simulink model "Supported_and_unsupported_combinations"  (Simulink 7.8)
settings: Solver=ode15s  StartTime=0.0  StopTime=inf  MaxStep=0.2  RelTol=1e-3
undefined symbols (not defined in the file): Engine, Engine1, Engine2, Engine3, Engine4, Engine5, Engine6, Engine7, Engine8, Engine9
libraries: sFunctionBlocks x32
(part 3 of 4)

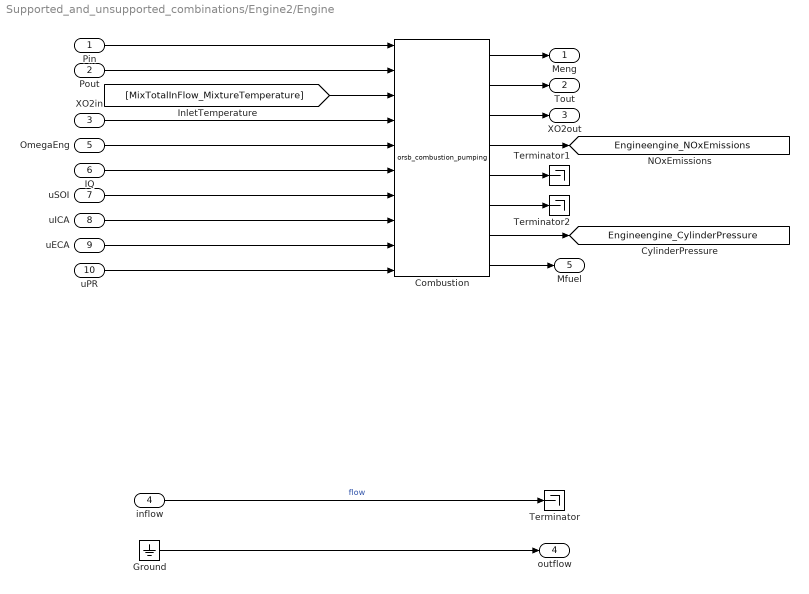
== system Supported_and_unsupported_combinations/Engine2/Engine ==
  Pin : Inport
  Pout : Inport  Port=2
  XO2in : Inport  Port=3
  inflow : Inport  Port=4
  OmegaEng : Inport  Port=5
  IQ : Inport  Port=6
  uSOI : Inport  Port=7
  uICA : Inport  Port=8
  uECA : Inport  Port=9
  uPR : Inport  Port=10
  Combustion : S-Function  FunctionName=orsb_combustion_pumping  Parameters=Displ, CompRatio, Ncyl, ValveMdl, TmpMdl, IgnitMdl, PressMdl, Cp, Cv, port_num_NOx, NOxMdl,  EnableBusSupport=off  mask(combustion_pumping){Displ=12.9, CompRatio=18, Ncyl=6, ValveMdl=[0.00961171539106083 -0.172384589641163], TmpMdl=[-0.025503095647334 0.175522235872159 0.0255043476751577 0.0373865335774022 0], IgnitMdl=[0.484351292851209 0.143524113288744 -0.055676015193126 -0.0109937044135945 -0.025686692856836], PressMdl=[5.48733176777509 -0.092135251339445 -0.0332005633970498 0.773921335537747], Cp=1500, Cv=1200, port_num_NOx=4, NOxMdl=[-0.0710772115732251 13.258266248882 2.53650929146028 -4.98871540780321 18.9690745540948 3.51983329140351 7.35640722696346 -29.5494146545499 -12.7663876549855 -0.0214097840965915 0.143608010417368 -1.21453634962735 0.541720620436424 -0.0774873942784366 -0.515304310267613]}
      mask prompts: Displ "displacement"; CompRatio "compression ratio"; Ncyl "number of cylinders"; ValveMdl "valve model"; TmpMdl "temperature model"; IgnitMdl "ignition model"; PressMdl "pressure model"; port_num_NOx "Model NOx output port number"; NOxMdl "NOx parameters"
      mask help: Combustion development
      mask TabNameString: geometry,geometry,geometry,thermodynamics,thermodynamics,thermodynamics,thermodynamics,thermodynamics,thermodynamics,NOx,NOx
      mask Display:
      | port_label('input', 1, 'Pi');
      | port_label('input', 2, 'Pe');
      | port_label('input', 3, 'Ti');
      | port_label('input', 4, 'O2i');
      | port_label('input', 5, 'Ne');
      | port_label('input', 6, 'iq');
      | port_label('input', 7, 'soi');
      | port_label('input', 8, 'ica');
      | port_label('input', 9, 'eca');
      | port_label('input', 10, 'Prail');
      | port_label('output', 1, 'M');
      | port_label('output', 2, 'Te');
      | port_label('output', 3, 'XO2e');
      | port_label('output', 4, 'NOx');
      | port_label('output', 5, 'lambda');
      | port_label('output', 6, 'phi_ign');
      | port_label('output', 7, 'Pcyl');
      | port_label('output', 8, 'Mf');
  Ground : Ground
  Terminator : Terminator
  Terminator1 : Terminator
  Terminator2 : Terminator
  Meng : Outport
  Tout : Outport  Port=2
  XO2out : Outport  Port=3
  outflow : Outport  Port=4
  Mfuel : Outport  Port=5
  tag scope: Engineengine_CylinderPressure=global, Engineengine_NOxEmissions=global
  wires:
  uSOI/1 -> Combustion/7
  [MixTotalInFlow_MixtureTemperature] -> Combustion/3
  Combustion/4 -> [Engineengine_NOxEmissions]
  XO2in/1 -> Combustion/4
  Combustion/3 -> XO2out/1
  Combustion/2 -> Tout/1
  Pout/1 -> Combustion/2
  Pin/1 -> Combustion/1
  OmegaEng/1 -> Combustion/5
  Ground/1 -> outflow/1
  inflow/1 -> Terminator/1  "flow"
  Combustion/1 -> Meng/1
  Combustion/5 -> Terminator1/1
  Combustion/6 -> Terminator2/1
  Combustion/7 -> [Engineengine_CylinderPressure]
  Combustion/8 -> Mfuel/1
  IQ/1 -> Combustion/6
  uICA/1 -> Combustion/8
  uECA/1 -> Combustion/9
  uPR/1 -> Combustion/10

== system Supported_and_unsupported_combinations/Engine2/ExhaustManifold ==
  Meng : Inport
  Tin : Inport  Port=2
  XO2in : Inport  Port=3
  inflow : Inport  Port=4
  Mfuel : Inport  Port=5
  Add4 : Sum
  AdiabaticManifoldXO2 : S-Function  FunctionName=orsb_reservoir_adiabatic_XO2  Parameters=V , R , Cp , pinit , Tinit , XO2init ,  EnableBusSupport=off  mask(reservoir adiabatic XO2 ){V=50, R=288.4, Cp=1135, pinit=247140, Tinit=720.22, XO2init=0.15}
      mask prompts: V "reservoir volume [l]"; R "gas constant [J/K/kg]"; Cp "fixed pressure spec heat [J/kg/K]"; pinit "initial pressure [Pa]"; Tinit "initial temperature [K]"; XO2init "initial oxygen mass fraction [-]"
      mask help: Adiabatic reservoir model with pressure, temperature, and oxygen mass fraction as internal states.
      mask TabNameString: General ,General ,General ,Initialization ,Initialization ,Initialization
      mask Display:
      | port_label('input', 1, 'min ');
      | port_label('input', 2, 'mout ');
      | port_label('input', 3, 'Tin ');
      | port_label('input', 4, 'O2min ');
      | port_label('output', 1, 'pout ');
      | port_label('output', 2, 'Tout ');
      | port_label('output', 3, 'XO2out ');
  Conversion_XO2_lambda : Fcn  Expr=u(1) / 0.231362 * (1 + 14.59) / (14.59 * (1 - u(1) / 0.231362))+1
  Product2 : Product  RndMeth=Zero
  Saturation : Saturate  UpperLimit=0.2313  LowerLimit=0
  Pout : Outport
  outflow : Outport  Port=2
  tag scope: EngineExhaustManifold_OutletLambda=global, EngineExhaustManifold_OutletOxygenFraction=global, EngineExhaustManifold_OutletPressure=global, EngineExhaustManifold_OutletTemperature=global
  wires:
  Conversion_XO2_lambda/1 -> [EngineExhaustManifold_OutletLambda]
  [FlowSplitterTotalOutFlow_Massflow] -> AdiabaticManifoldXO2/2
  Mfuel/1 -> Add4/1
  inflow/1 -> outflow/1  "flow"
  XO2in/1 -> Product2/2
  AdiabaticManifoldXO2/3 -> [EngineExhaustManifold_OutletOxygenFraction], Saturation/1
  Tin/1 -> AdiabaticManifoldXO2/3
  AdiabaticManifoldXO2/2 -> [EngineExhaustManifold_OutletTemperature]
  AdiabaticManifoldXO2/1 -> [EngineExhaustManifold_OutletPressure], Pout/1
  Meng/1 -> Add4/2
  Product2/1 -> AdiabaticManifoldXO2/4
  Add4/1 -> Product2/1, AdiabaticManifoldXO2/1
  Saturation/1 -> Conversion_XO2_lambda/1

== system Supported_and_unsupported_combinations/Engine2/IntakeManifold ==
  Mout : Inport
  inflow : Inport  Port=2
  IsothermalManifoldXO2 : S-Function  FunctionName=orsb_reservoir_isothermal_XO2  Parameters=V , R , Cp , pinit , XO2init ,  EnableBusSupport=off  mask(reservoir isothermal XO2 ){V=41.2801, R=288.4, Cp=1020, pinit=205590, XO2init=0.22}
      mask prompts: V "reservoir volume [l]"; R "gas constant [J/K/kg]"; Cp "fixed pressure spec heat [J/kg/K]"; pinit "initial pressure [Pa]"; XO2init "initial oxygen mass fraction [-]"
      mask help: Isothermal reservoir model with pressure and oxygen mass fraction as internal states.
      mask TabNameString: General ,General ,General ,Initialization ,Initialization
      mask Display:
      | port_label('input', 1, 'min ');
      | port_label('input', 2, 'mout ');
      | port_label('input', 3, 'Tin ');
      | port_label('input', 4, 'O2min ');
      | port_label('output', 1, 'pout ');
      | port_label('output', 2, 'XO2out ');
  Pim : Outport
  XO2out : Outport  Port=2
  outflow : Outport  Port=3
  tag scope: EngineIntakeManifold_OutletPressure=global
  wires:
  [MixTotalInFlow_MixtureTemperature] -> IsothermalManifoldXO2/3
  [MixTotalInFlow_OxygenFlow] -> IsothermalManifoldXO2/4
  [MixTotalInFlow_Massflow] -> IsothermalManifoldXO2/1
  inflow/1 -> outflow/1  "flow"
  IsothermalManifoldXO2/2 -> XO2out/1
  IsothermalManifoldXO2/1 -> [EngineIntakeManifold_OutletPressure], Pim/1
  Mout/1 -> IsothermalManifoldXO2/2

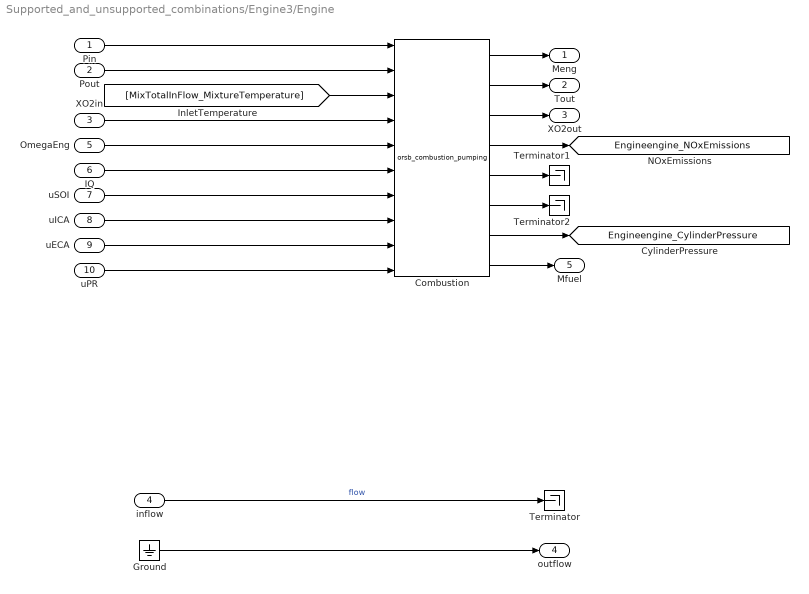
== system Supported_and_unsupported_combinations/Engine3/Engine ==
  Pin : Inport
  Pout : Inport  Port=2
  XO2in : Inport  Port=3
  inflow : Inport  Port=4
  OmegaEng : Inport  Port=5
  IQ : Inport  Port=6
  uSOI : Inport  Port=7
  uICA : Inport  Port=8
  uECA : Inport  Port=9
  uPR : Inport  Port=10
  Combustion : S-Function  FunctionName=orsb_combustion_pumping  Parameters=Displ, CompRatio, Ncyl, ValveMdl, TmpMdl, IgnitMdl, PressMdl, Cp, Cv, port_num_NOx, NOxMdl,  EnableBusSupport=off  mask(combustion_pumping){Displ=12.9, CompRatio=18, Ncyl=6, ValveMdl=[0.00961171539106083 -0.172384589641163], TmpMdl=[-0.025503095647334 0.175522235872159 0.0255043476751577 0.0373865335774022 0], IgnitMdl=[0.484351292851209 0.143524113288744 -0.055676015193126 -0.0109937044135945 -0.025686692856836], PressMdl=[5.48733176777509 -0.092135251339445 -0.0332005633970498 0.773921335537747], Cp=1500, Cv=1200, port_num_NOx=4, NOxMdl=[-0.0710772115732251 13.258266248882 2.53650929146028 -4.98871540780321 18.9690745540948 3.51983329140351 7.35640722696346 -29.5494146545499 -12.7663876549855 -0.0214097840965915 0.143608010417368 -1.21453634962735 0.541720620436424 -0.0774873942784366 -0.515304310267613]}
      mask prompts: Displ "displacement"; CompRatio "compression ratio"; Ncyl "number of cylinders"; ValveMdl "valve model"; TmpMdl "temperature model"; IgnitMdl "ignition model"; PressMdl "pressure model"; port_num_NOx "Model NOx output port number"; NOxMdl "NOx parameters"
      mask help: Combustion development
      mask TabNameString: geometry,geometry,geometry,thermodynamics,thermodynamics,thermodynamics,thermodynamics,thermodynamics,thermodynamics,NOx,NOx
      mask Display:
      | port_label('input', 1, 'Pi');
      | port_label('input', 2, 'Pe');
      | port_label('input', 3, 'Ti');
      | port_label('input', 4, 'O2i');
      | port_label('input', 5, 'Ne');
      | port_label('input', 6, 'iq');
      | port_label('input', 7, 'soi');
      | port_label('input', 8, 'ica');
      | port_label('input', 9, 'eca');
      | port_label('input', 10, 'Prail');
      | port_label('output', 1, 'M');
      | port_label('output', 2, 'Te');
      | port_label('output', 3, 'XO2e');
      | port_label('output', 4, 'NOx');
      | port_label('output', 5, 'lambda');
      | port_label('output', 6, 'phi_ign');
      | port_label('output', 7, 'Pcyl');
      | port_label('output', 8, 'Mf');
  Ground : Ground
  Terminator : Terminator
  Terminator1 : Terminator
  Terminator2 : Terminator
  Meng : Outport
  Tout : Outport  Port=2
  XO2out : Outport  Port=3
  outflow : Outport  Port=4
  Mfuel : Outport  Port=5
  tag scope: Engineengine_CylinderPressure=global, Engineengine_NOxEmissions=global
  wires:
  uPR/1 -> Combustion/10
  uECA/1 -> Combustion/9
  uICA/1 -> Combustion/8
  IQ/1 -> Combustion/6
  Combustion/8 -> Mfuel/1
  Combustion/7 -> [Engineengine_CylinderPressure]
  Combustion/6 -> Terminator2/1
  Combustion/5 -> Terminator1/1
  Combustion/1 -> Meng/1
  inflow/1 -> Terminator/1  "flow"
  Ground/1 -> outflow/1
  OmegaEng/1 -> Combustion/5
  Pin/1 -> Combustion/1
  Pout/1 -> Combustion/2
  Combustion/2 -> Tout/1
  Combustion/3 -> XO2out/1
  XO2in/1 -> Combustion/4
  Combustion/4 -> [Engineengine_NOxEmissions]
  [MixTotalInFlow_MixtureTemperature] -> Combustion/3
  uSOI/1 -> Combustion/7

== system Supported_and_unsupported_combinations/Engine3/ExhaustManifold ==
  Meng : Inport
  Tin : Inport  Port=2
  XO2in : Inport  Port=3
  inflow : Inport  Port=4
  Mfuel : Inport  Port=5
  Add4 : Sum
  AdiabaticManifoldXO2 : S-Function  FunctionName=orsb_reservoir_adiabatic_XO2  Parameters=V , R , Cp , pinit , Tinit , XO2init ,  EnableBusSupport=off  mask(reservoir adiabatic XO2 ){V=50, R=288.4, Cp=1135, pinit=247140, Tinit=720.22, XO2init=0.15}
      mask prompts: V "reservoir volume [l]"; R "gas constant [J/K/kg]"; Cp "fixed pressure spec heat [J/kg/K]"; pinit "initial pressure [Pa]"; Tinit "initial temperature [K]"; XO2init "initial oxygen mass fraction [-]"
      mask help: Adiabatic reservoir model with pressure, temperature, and oxygen mass fraction as internal states.
      mask TabNameString: General ,General ,General ,Initialization ,Initialization ,Initialization
      mask Display:
      | port_label('input', 1, 'min ');
      | port_label('input', 2, 'mout ');
      | port_label('input', 3, 'Tin ');
      | port_label('input', 4, 'O2min ');
      | port_label('output', 1, 'pout ');
      | port_label('output', 2, 'Tout ');
      | port_label('output', 3, 'XO2out ');
  Conversion_XO2_lambda : Fcn  Expr=u(1) / 0.231362 * (1 + 14.59) / (14.59 * (1 - u(1) / 0.231362))+1
  Product2 : Product  RndMeth=Zero
  Saturation : Saturate  UpperLimit=0.2313  LowerLimit=0
  Pout : Outport
  outflow : Outport  Port=2
  tag scope: EngineExhaustManifold_OutletLambda=global, EngineExhaustManifold_OutletOxygenFraction=global, EngineExhaustManifold_OutletPressure=global, EngineExhaustManifold_OutletTemperature=global
  wires:
  Saturation/1 -> Conversion_XO2_lambda/1
  Add4/1 -> AdiabaticManifoldXO2/1, Product2/1
  Product2/1 -> AdiabaticManifoldXO2/4
  Meng/1 -> Add4/2
  AdiabaticManifoldXO2/1 -> Pout/1, [EngineExhaustManifold_OutletPressure]
  AdiabaticManifoldXO2/2 -> [EngineExhaustManifold_OutletTemperature]
  Tin/1 -> AdiabaticManifoldXO2/3
  AdiabaticManifoldXO2/3 -> Saturation/1, [EngineExhaustManifold_OutletOxygenFraction]
  XO2in/1 -> Product2/2
  inflow/1 -> outflow/1  "flow"
  Mfuel/1 -> Add4/1
  [FlowSplitterTotalOutFlow_Massflow] -> AdiabaticManifoldXO2/2
  Conversion_XO2_lambda/1 -> [EngineExhaustManifold_OutletLambda]

== system Supported_and_unsupported_combinations/Engine3/IntakeManifold ==
  Mout : Inport
  inflow : Inport  Port=2
  IsothermalManifoldXO2 : S-Function  FunctionName=orsb_reservoir_isothermal_XO2  Parameters=V , R , Cp , pinit , XO2init ,  EnableBusSupport=off  mask(reservoir isothermal XO2 ){V=41.2801, R=288.4, Cp=1020, pinit=205590, XO2init=0.22}
      mask prompts: V "reservoir volume [l]"; R "gas constant [J/K/kg]"; Cp "fixed pressure spec heat [J/kg/K]"; pinit "initial pressure [Pa]"; XO2init "initial oxygen mass fraction [-]"
      mask help: Isothermal reservoir model with pressure and oxygen mass fraction as internal states.
      mask TabNameString: General ,General ,General ,Initialization ,Initialization
      mask Display:
      | port_label('input', 1, 'min ');
      | port_label('input', 2, 'mout ');
      | port_label('input', 3, 'Tin ');
      | port_label('input', 4, 'O2min ');
      | port_label('output', 1, 'pout ');
      | port_label('output', 2, 'XO2out ');
  Pim : Outport
  XO2out : Outport  Port=2
  outflow : Outport  Port=3
  tag scope: EngineIntakeManifold_OutletPressure=global
  wires:
  Mout/1 -> IsothermalManifoldXO2/2
  IsothermalManifoldXO2/1 -> Pim/1, [EngineIntakeManifold_OutletPressure]
  IsothermalManifoldXO2/2 -> XO2out/1
  inflow/1 -> outflow/1  "flow"
  [MixTotalInFlow_Massflow] -> IsothermalManifoldXO2/1
  [MixTotalInFlow_OxygenFlow] -> IsothermalManifoldXO2/4
  [MixTotalInFlow_MixtureTemperature] -> IsothermalManifoldXO2/3

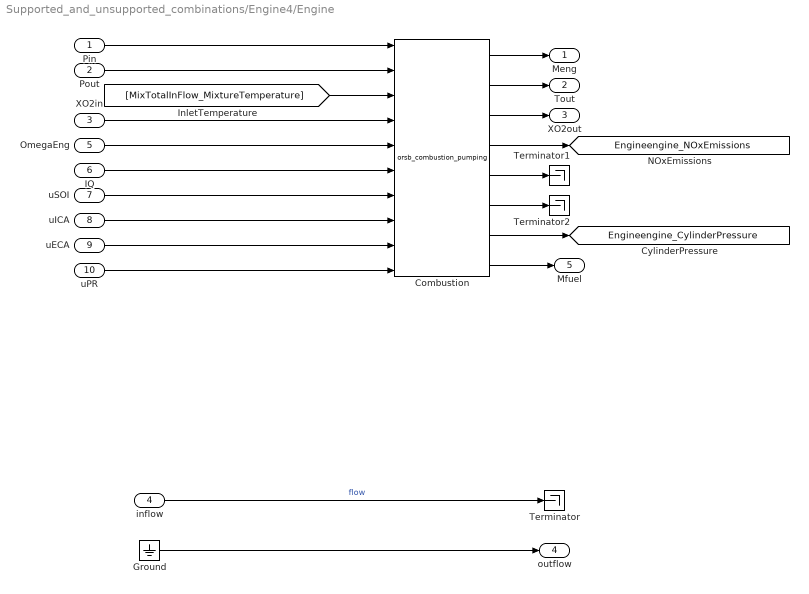
== system Supported_and_unsupported_combinations/Engine4/Engine ==
  Pin : Inport
  Pout : Inport  Port=2
  XO2in : Inport  Port=3
  inflow : Inport  Port=4
  OmegaEng : Inport  Port=5
  IQ : Inport  Port=6
  uSOI : Inport  Port=7
  uICA : Inport  Port=8
  uECA : Inport  Port=9
  uPR : Inport  Port=10
  Combustion : S-Function  FunctionName=orsb_combustion_pumping  Parameters=Displ, CompRatio, Ncyl, ValveMdl, TmpMdl, IgnitMdl, PressMdl, Cp, Cv, port_num_NOx, NOxMdl,  EnableBusSupport=off  mask(combustion_pumping){Displ=12.9, CompRatio=18, Ncyl=6, ValveMdl=[0.00961171539106083 -0.172384589641163], TmpMdl=[-0.025503095647334 0.175522235872159 0.0255043476751577 0.0373865335774022 0], IgnitMdl=[0.484351292851209 0.143524113288744 -0.055676015193126 -0.0109937044135945 -0.025686692856836], PressMdl=[5.48733176777509 -0.092135251339445 -0.0332005633970498 0.773921335537747], Cp=1500, Cv=1200, port_num_NOx=4, NOxMdl=[-0.0710772115732251 13.258266248882 2.53650929146028 -4.98871540780321 18.9690745540948 3.51983329140351 7.35640722696346 -29.5494146545499 -12.7663876549855 -0.0214097840965915 0.143608010417368 -1.21453634962735 0.541720620436424 -0.0774873942784366 -0.515304310267613]}
      mask prompts: Displ "displacement"; CompRatio "compression ratio"; Ncyl "number of cylinders"; ValveMdl "valve model"; TmpMdl "temperature model"; IgnitMdl "ignition model"; PressMdl "pressure model"; port_num_NOx "Model NOx output port number"; NOxMdl "NOx parameters"
      mask help: Combustion development
      mask TabNameString: geometry,geometry,geometry,thermodynamics,thermodynamics,thermodynamics,thermodynamics,thermodynamics,thermodynamics,NOx,NOx
      mask Display:
      | port_label('input', 1, 'Pi');
      | port_label('input', 2, 'Pe');
      | port_label('input', 3, 'Ti');
      | port_label('input', 4, 'O2i');
      | port_label('input', 5, 'Ne');
      | port_label('input', 6, 'iq');
      | port_label('input', 7, 'soi');
      | port_label('input', 8, 'ica');
      | port_label('input', 9, 'eca');
      | port_label('input', 10, 'Prail');
      | port_label('output', 1, 'M');
      | port_label('output', 2, 'Te');
      | port_label('output', 3, 'XO2e');
      | port_label('output', 4, 'NOx');
      | port_label('output', 5, 'lambda');
      | port_label('output', 6, 'phi_ign');
      | port_label('output', 7, 'Pcyl');
      | port_label('output', 8, 'Mf');
  Ground : Ground
  Terminator : Terminator
  Terminator1 : Terminator
  Terminator2 : Terminator
  Meng : Outport
  Tout : Outport  Port=2
  XO2out : Outport  Port=3
  outflow : Outport  Port=4
  Mfuel : Outport  Port=5
  tag scope: Engineengine_CylinderPressure=global, Engineengine_NOxEmissions=global
  wires:
  uSOI/1 -> Combustion/7
  [MixTotalInFlow_MixtureTemperature] -> Combustion/3
  Combustion/4 -> [Engineengine_NOxEmissions]
  XO2in/1 -> Combustion/4
  Combustion/3 -> XO2out/1
  Combustion/2 -> Tout/1
  Pout/1 -> Combustion/2
  Pin/1 -> Combustion/1
  OmegaEng/1 -> Combustion/5
  Ground/1 -> outflow/1
  inflow/1 -> Terminator/1  "flow"
  Combustion/1 -> Meng/1
  Combustion/5 -> Terminator1/1
  Combustion/6 -> Terminator2/1
  Combustion/7 -> [Engineengine_CylinderPressure]
  Combustion/8 -> Mfuel/1
  IQ/1 -> Combustion/6
  uICA/1 -> Combustion/8
  uECA/1 -> Combustion/9
  uPR/1 -> Combustion/10

== system Supported_and_unsupported_combinations/Engine4/ExhaustManifold ==
  Meng : Inport
  Tin : Inport  Port=2
  XO2in : Inport  Port=3
  inflow : Inport  Port=4
  Mfuel : Inport  Port=5
  Add4 : Sum
  AdiabaticManifoldXO2 : S-Function  FunctionName=orsb_reservoir_adiabatic_XO2  Parameters=V , R , Cp , pinit , Tinit , XO2init ,  EnableBusSupport=off  mask(reservoir adiabatic XO2 ){V=50, R=288.4, Cp=1135, pinit=247140, Tinit=720.22, XO2init=0.15}
      mask prompts: V "reservoir volume [l]"; R "gas constant [J/K/kg]"; Cp "fixed pressure spec heat [J/kg/K]"; pinit "initial pressure [Pa]"; Tinit "initial temperature [K]"; XO2init "initial oxygen mass fraction [-]"
      mask help: Adiabatic reservoir model with pressure, temperature, and oxygen mass fraction as internal states.
      mask TabNameString: General ,General ,General ,Initialization ,Initialization ,Initialization
      mask Display:
      | port_label('input', 1, 'min ');
      | port_label('input', 2, 'mout ');
      | port_label('input', 3, 'Tin ');
      | port_label('input', 4, 'O2min ');
      | port_label('output', 1, 'pout ');
      | port_label('output', 2, 'Tout ');
      | port_label('output', 3, 'XO2out ');
  Conversion_XO2_lambda : Fcn  Expr=u(1) / 0.231362 * (1 + 14.59) / (14.59 * (1 - u(1) / 0.231362))+1
  Product2 : Product  RndMeth=Zero
  Saturation : Saturate  UpperLimit=0.2313  LowerLimit=0
  Pout : Outport
  outflow : Outport  Port=2
  tag scope: EngineExhaustManifold_OutletLambda=global, EngineExhaustManifold_OutletOxygenFraction=global, EngineExhaustManifold_OutletPressure=global, EngineExhaustManifold_OutletTemperature=global
  wires:
  Conversion_XO2_lambda/1 -> [EngineExhaustManifold_OutletLambda]
  [FlowSplitterTotalOutFlow_Massflow] -> AdiabaticManifoldXO2/2
  Mfuel/1 -> Add4/1
  inflow/1 -> outflow/1  "flow"
  XO2in/1 -> Product2/2
  AdiabaticManifoldXO2/3 -> [EngineExhaustManifold_OutletOxygenFraction], Saturation/1
  Tin/1 -> AdiabaticManifoldXO2/3
  AdiabaticManifoldXO2/2 -> [EngineExhaustManifold_OutletTemperature]
  AdiabaticManifoldXO2/1 -> [EngineExhaustManifold_OutletPressure], Pout/1
  Meng/1 -> Add4/2
  Product2/1 -> AdiabaticManifoldXO2/4
  Add4/1 -> Product2/1, AdiabaticManifoldXO2/1
  Saturation/1 -> Conversion_XO2_lambda/1

== system Supported_and_unsupported_combinations/Engine4/IntakeManifold ==
  Mout : Inport
  inflow : Inport  Port=2
  IsothermalManifoldXO2 : S-Function  FunctionName=orsb_reservoir_isothermal_XO2  Parameters=V , R , Cp , pinit , XO2init ,  EnableBusSupport=off  mask(reservoir isothermal XO2 ){V=41.2801, R=288.4, Cp=1020, pinit=205590, XO2init=0.22}
      mask prompts: V "reservoir volume [l]"; R "gas constant [J/K/kg]"; Cp "fixed pressure spec heat [J/kg/K]"; pinit "initial pressure [Pa]"; XO2init "initial oxygen mass fraction [-]"
      mask help: Isothermal reservoir model with pressure and oxygen mass fraction as internal states.
      mask TabNameString: General ,General ,General ,Initialization ,Initialization
      mask Display:
      | port_label('input', 1, 'min ');
      | port_label('input', 2, 'mout ');
      | port_label('input', 3, 'Tin ');
      | port_label('input', 4, 'O2min ');
      | port_label('output', 1, 'pout ');
      | port_label('output', 2, 'XO2out ');
  Pim : Outport
  XO2out : Outport  Port=2
  outflow : Outport  Port=3
  tag scope: EngineIntakeManifold_OutletPressure=global
  wires:
  [MixTotalInFlow_MixtureTemperature] -> IsothermalManifoldXO2/3
  [MixTotalInFlow_OxygenFlow] -> IsothermalManifoldXO2/4
  [MixTotalInFlow_Massflow] -> IsothermalManifoldXO2/1
  inflow/1 -> outflow/1  "flow"
  IsothermalManifoldXO2/2 -> XO2out/1
  IsothermalManifoldXO2/1 -> [EngineIntakeManifold_OutletPressure], Pim/1
  Mout/1 -> IsothermalManifoldXO2/2

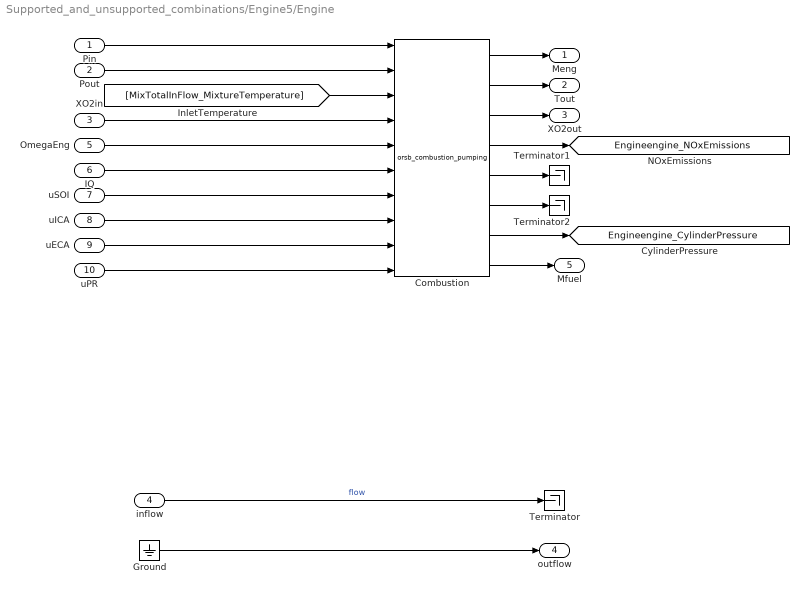
== system Supported_and_unsupported_combinations/Engine5/Engine ==
  Pin : Inport
  Pout : Inport  Port=2
  XO2in : Inport  Port=3
  inflow : Inport  Port=4
  OmegaEng : Inport  Port=5
  IQ : Inport  Port=6
  uSOI : Inport  Port=7
  uICA : Inport  Port=8
  uECA : Inport  Port=9
  uPR : Inport  Port=10
  Combustion : S-Function  FunctionName=orsb_combustion_pumping  Parameters=Displ, CompRatio, Ncyl, ValveMdl, TmpMdl, IgnitMdl, PressMdl, Cp, Cv, port_num_NOx, NOxMdl,  EnableBusSupport=off  mask(combustion_pumping){Displ=12.9, CompRatio=18, Ncyl=6, ValveMdl=[0.00961171539106083 -0.172384589641163], TmpMdl=[-0.025503095647334 0.175522235872159 0.0255043476751577 0.0373865335774022 0], IgnitMdl=[0.484351292851209 0.143524113288744 -0.055676015193126 -0.0109937044135945 -0.025686692856836], PressMdl=[5.48733176777509 -0.092135251339445 -0.0332005633970498 0.773921335537747], Cp=1500, Cv=1200, port_num_NOx=4, NOxMdl=[-0.0710772115732251 13.258266248882 2.53650929146028 -4.98871540780321 18.9690745540948 3.51983329140351 7.35640722696346 -29.5494146545499 -12.7663876549855 -0.0214097840965915 0.143608010417368 -1.21453634962735 0.541720620436424 -0.0774873942784366 -0.515304310267613]}
      mask prompts: Displ "displacement"; CompRatio "compression ratio"; Ncyl "number of cylinders"; ValveMdl "valve model"; TmpMdl "temperature model"; IgnitMdl "ignition model"; PressMdl "pressure model"; port_num_NOx "Model NOx output port number"; NOxMdl "NOx parameters"
      mask help: Combustion development
      mask TabNameString: geometry,geometry,geometry,thermodynamics,thermodynamics,thermodynamics,thermodynamics,thermodynamics,thermodynamics,NOx,NOx
      mask Display:
      | port_label('input', 1, 'Pi');
      | port_label('input', 2, 'Pe');
      | port_label('input', 3, 'Ti');
      | port_label('input', 4, 'O2i');
      | port_label('input', 5, 'Ne');
      | port_label('input', 6, 'iq');
      | port_label('input', 7, 'soi');
      | port_label('input', 8, 'ica');
      | port_label('input', 9, 'eca');
      | port_label('input', 10, 'Prail');
      | port_label('output', 1, 'M');
      | port_label('output', 2, 'Te');
      | port_label('output', 3, 'XO2e');
      | port_label('output', 4, 'NOx');
      | port_label('output', 5, 'lambda');
      | port_label('output', 6, 'phi_ign');
      | port_label('output', 7, 'Pcyl');
      | port_label('output', 8, 'Mf');
  Ground : Ground
  Terminator : Terminator
  Terminator1 : Terminator
  Terminator2 : Terminator
  Meng : Outport
  Tout : Outport  Port=2
  XO2out : Outport  Port=3
  outflow : Outport  Port=4
  Mfuel : Outport  Port=5
  tag scope: Engineengine_CylinderPressure=global, Engineengine_NOxEmissions=global
  wires:
  uPR/1 -> Combustion/10
  uECA/1 -> Combustion/9
  uICA/1 -> Combustion/8
  IQ/1 -> Combustion/6
  Combustion/8 -> Mfuel/1
  Combustion/7 -> [Engineengine_CylinderPressure]
  Combustion/6 -> Terminator2/1
  Combustion/5 -> Terminator1/1
  Combustion/1 -> Meng/1
  inflow/1 -> Terminator/1  "flow"
  Ground/1 -> outflow/1
  OmegaEng/1 -> Combustion/5
  Pin/1 -> Combustion/1
  Pout/1 -> Combustion/2
  Combustion/2 -> Tout/1
  Combustion/3 -> XO2out/1
  XO2in/1 -> Combustion/4
  Combustion/4 -> [Engineengine_NOxEmissions]
  [MixTotalInFlow_MixtureTemperature] -> Combustion/3
  uSOI/1 -> Combustion/7

== system Supported_and_unsupported_combinations/Engine5/ExhaustManifold ==
  Meng : Inport
  Tin : Inport  Port=2
  XO2in : Inport  Port=3
  inflow : Inport  Port=4
  Mfuel : Inport  Port=5
  Add4 : Sum
  AdiabaticManifoldXO2 : S-Function  FunctionName=orsb_reservoir_adiabatic_XO2  Parameters=V , R , Cp , pinit , Tinit , XO2init ,  EnableBusSupport=off  mask(reservoir adiabatic XO2 ){V=50, R=288.4, Cp=1135, pinit=247140, Tinit=720.22, XO2init=0.15}
      mask prompts: V "reservoir volume [l]"; R "gas constant [J/K/kg]"; Cp "fixed pressure spec heat [J/kg/K]"; pinit "initial pressure [Pa]"; Tinit "initial temperature [K]"; XO2init "initial oxygen mass fraction [-]"
      mask help: Adiabatic reservoir model with pressure, temperature, and oxygen mass fraction as internal states.
      mask TabNameString: General ,General ,General ,Initialization ,Initialization ,Initialization
      mask Display:
      | port_label('input', 1, 'min ');
      | port_label('input', 2, 'mout ');
      | port_label('input', 3, 'Tin ');
      | port_label('input', 4, 'O2min ');
      | port_label('output', 1, 'pout ');
      | port_label('output', 2, 'Tout ');
      | port_label('output', 3, 'XO2out ');
  Conversion_XO2_lambda : Fcn  Expr=u(1) / 0.231362 * (1 + 14.59) / (14.59 * (1 - u(1) / 0.231362))+1
  Product2 : Product  RndMeth=Zero
  Saturation : Saturate  UpperLimit=0.2313  LowerLimit=0
  Pout : Outport
  outflow : Outport  Port=2
  tag scope: EngineExhaustManifold_OutletLambda=global, EngineExhaustManifold_OutletOxygenFraction=global, EngineExhaustManifold_OutletPressure=global, EngineExhaustManifold_OutletTemperature=global
  wires:
  Saturation/1 -> Conversion_XO2_lambda/1
  Add4/1 -> AdiabaticManifoldXO2/1, Product2/1
  Product2/1 -> AdiabaticManifoldXO2/4
  Meng/1 -> Add4/2
  AdiabaticManifoldXO2/1 -> Pout/1, [EngineExhaustManifold_OutletPressure]
  AdiabaticManifoldXO2/2 -> [EngineExhaustManifold_OutletTemperature]
  Tin/1 -> AdiabaticManifoldXO2/3
  AdiabaticManifoldXO2/3 -> Saturation/1, [EngineExhaustManifold_OutletOxygenFraction]
  XO2in/1 -> Product2/2
  inflow/1 -> outflow/1  "flow"
  Mfuel/1 -> Add4/1
  [FlowSplitterTotalOutFlow_Massflow] -> AdiabaticManifoldXO2/2
  Conversion_XO2_lambda/1 -> [EngineExhaustManifold_OutletLambda]

== system Supported_and_unsupported_combinations/Engine5/IntakeManifold ==
  Mout : Inport
  inflow : Inport  Port=2
  IsothermalManifoldXO2 : S-Function  FunctionName=orsb_reservoir_isothermal_XO2  Parameters=V , R , Cp , pinit , XO2init ,  EnableBusSupport=off  mask(reservoir isothermal XO2 ){V=41.2801, R=288.4, Cp=1020, pinit=205590, XO2init=0.22}
      mask prompts: V "reservoir volume [l]"; R "gas constant [J/K/kg]"; Cp "fixed pressure spec heat [J/kg/K]"; pinit "initial pressure [Pa]"; XO2init "initial oxygen mass fraction [-]"
      mask help: Isothermal reservoir model with pressure and oxygen mass fraction as internal states.
      mask TabNameString: General ,General ,General ,Initialization ,Initialization
      mask Display:
      | port_label('input', 1, 'min ');
      | port_label('input', 2, 'mout ');
      | port_label('input', 3, 'Tin ');
      | port_label('input', 4, 'O2min ');
      | port_label('output', 1, 'pout ');
      | port_label('output', 2, 'XO2out ');
  Pim : Outport
  XO2out : Outport  Port=2
  outflow : Outport  Port=3
  tag scope: EngineIntakeManifold_OutletPressure=global
  wires:
  Mout/1 -> IsothermalManifoldXO2/2
  IsothermalManifoldXO2/1 -> Pim/1, [EngineIntakeManifold_OutletPressure]
  IsothermalManifoldXO2/2 -> XO2out/1
  inflow/1 -> outflow/1  "flow"
  [MixTotalInFlow_Massflow] -> IsothermalManifoldXO2/1
  [MixTotalInFlow_OxygenFlow] -> IsothermalManifoldXO2/4
  [MixTotalInFlow_MixtureTemperature] -> IsothermalManifoldXO2/3

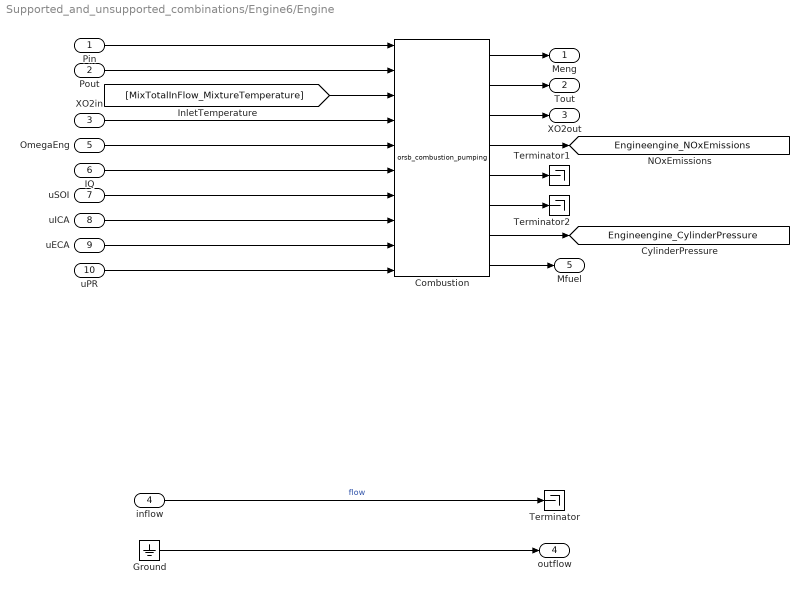
== system Supported_and_unsupported_combinations/Engine6/Engine ==
  Pin : Inport
  Pout : Inport  Port=2
  XO2in : Inport  Port=3
  inflow : Inport  Port=4
  OmegaEng : Inport  Port=5
  IQ : Inport  Port=6
  uSOI : Inport  Port=7
  uICA : Inport  Port=8
  uECA : Inport  Port=9
  uPR : Inport  Port=10
  Combustion : S-Function  FunctionName=orsb_combustion_pumping  Parameters=Displ, CompRatio, Ncyl, ValveMdl, TmpMdl, IgnitMdl, PressMdl, Cp, Cv, port_num_NOx, NOxMdl,  EnableBusSupport=off  mask(combustion_pumping){Displ=12.9, CompRatio=18, Ncyl=6, ValveMdl=[0.00961171539106083 -0.172384589641163], TmpMdl=[-0.025503095647334 0.175522235872159 0.0255043476751577 0.0373865335774022 0], IgnitMdl=[0.484351292851209 0.143524113288744 -0.055676015193126 -0.0109937044135945 -0.025686692856836], PressMdl=[5.48733176777509 -0.092135251339445 -0.0332005633970498 0.773921335537747], Cp=1500, Cv=1200, port_num_NOx=4, NOxMdl=[-0.0710772115732251 13.258266248882 2.53650929146028 -4.98871540780321 18.9690745540948 3.51983329140351 7.35640722696346 -29.5494146545499 -12.7663876549855 -0.0214097840965915 0.143608010417368 -1.21453634962735 0.541720620436424 -0.0774873942784366 -0.515304310267613]}
      mask prompts: Displ "displacement"; CompRatio "compression ratio"; Ncyl "number of cylinders"; ValveMdl "valve model"; TmpMdl "temperature model"; IgnitMdl "ignition model"; PressMdl "pressure model"; port_num_NOx "Model NOx output port number"; NOxMdl "NOx parameters"
      mask help: Combustion development
      mask TabNameString: geometry,geometry,geometry,thermodynamics,thermodynamics,thermodynamics,thermodynamics,thermodynamics,thermodynamics,NOx,NOx
      mask Display:
      | port_label('input', 1, 'Pi');
      | port_label('input', 2, 'Pe');
      | port_label('input', 3, 'Ti');
      | port_label('input', 4, 'O2i');
      | port_label('input', 5, 'Ne');
      | port_label('input', 6, 'iq');
      | port_label('input', 7, 'soi');
      | port_label('input', 8, 'ica');
      | port_label('input', 9, 'eca');
      | port_label('input', 10, 'Prail');
      | port_label('output', 1, 'M');
      | port_label('output', 2, 'Te');
      | port_label('output', 3, 'XO2e');
      | port_label('output', 4, 'NOx');
      | port_label('output', 5, 'lambda');
      | port_label('output', 6, 'phi_ign');
      | port_label('output', 7, 'Pcyl');
      | port_label('output', 8, 'Mf');
  Ground : Ground
  Terminator : Terminator
  Terminator1 : Terminator
  Terminator2 : Terminator
  Meng : Outport
  Tout : Outport  Port=2
  XO2out : Outport  Port=3
  outflow : Outport  Port=4
  Mfuel : Outport  Port=5
  tag scope: Engineengine_CylinderPressure=global, Engineengine_NOxEmissions=global
  wires:
  uPR/1 -> Combustion/10
  uECA/1 -> Combustion/9
  uICA/1 -> Combustion/8
  IQ/1 -> Combustion/6
  Combustion/8 -> Mfuel/1
  Combustion/7 -> [Engineengine_CylinderPressure]
  Combustion/6 -> Terminator2/1
  Combustion/5 -> Terminator1/1
  Combustion/1 -> Meng/1
  inflow/1 -> Terminator/1  "flow"
  Ground/1 -> outflow/1
  OmegaEng/1 -> Combustion/5
  Pin/1 -> Combustion/1
  Pout/1 -> Combustion/2
  Combustion/2 -> Tout/1
  Combustion/3 -> XO2out/1
  XO2in/1 -> Combustion/4
  Combustion/4 -> [Engineengine_NOxEmissions]
  [MixTotalInFlow_MixtureTemperature] -> Combustion/3
  uSOI/1 -> Combustion/7

== system Supported_and_unsupported_combinations/Engine6/ExhaustManifold ==
  Meng : Inport
  Tin : Inport  Port=2
  XO2in : Inport  Port=3
  inflow : Inport  Port=4
  Mfuel : Inport  Port=5
  Add4 : Sum
  AdiabaticManifoldXO2 : S-Function  FunctionName=orsb_reservoir_adiabatic_XO2  Parameters=V , R , Cp , pinit , Tinit , XO2init ,  EnableBusSupport=off  mask(reservoir adiabatic XO2 ){V=50, R=288.4, Cp=1135, pinit=247140, Tinit=720.22, XO2init=0.15}
      mask prompts: V "reservoir volume [l]"; R "gas constant [J/K/kg]"; Cp "fixed pressure spec heat [J/kg/K]"; pinit "initial pressure [Pa]"; Tinit "initial temperature [K]"; XO2init "initial oxygen mass fraction [-]"
      mask help: Adiabatic reservoir model with pressure, temperature, and oxygen mass fraction as internal states.
      mask TabNameString: General ,General ,General ,Initialization ,Initialization ,Initialization
      mask Display:
      | port_label('input', 1, 'min ');
      | port_label('input', 2, 'mout ');
      | port_label('input', 3, 'Tin ');
      | port_label('input', 4, 'O2min ');
      | port_label('output', 1, 'pout ');
      | port_label('output', 2, 'Tout ');
      | port_label('output', 3, 'XO2out ');
  Conversion_XO2_lambda : Fcn  Expr=u(1) / 0.231362 * (1 + 14.59) / (14.59 * (1 - u(1) / 0.231362))+1
  Product2 : Product  RndMeth=Zero
  Saturation : Saturate  UpperLimit=0.2313  LowerLimit=0
  Pout : Outport
  outflow : Outport  Port=2
  tag scope: EngineExhaustManifold_OutletLambda=global, EngineExhaustManifold_OutletOxygenFraction=global, EngineExhaustManifold_OutletPressure=global, EngineExhaustManifold_OutletTemperature=global
  wires:
  Saturation/1 -> Conversion_XO2_lambda/1
  Add4/1 -> AdiabaticManifoldXO2/1, Product2/1
  Product2/1 -> AdiabaticManifoldXO2/4
  Meng/1 -> Add4/2
  AdiabaticManifoldXO2/1 -> Pout/1, [EngineExhaustManifold_OutletPressure]
  AdiabaticManifoldXO2/2 -> [EngineExhaustManifold_OutletTemperature]
  Tin/1 -> AdiabaticManifoldXO2/3
  AdiabaticManifoldXO2/3 -> Saturation/1, [EngineExhaustManifold_OutletOxygenFraction]
  XO2in/1 -> Product2/2
  inflow/1 -> outflow/1  "flow"
  Mfuel/1 -> Add4/1
  [FlowSplitterTotalOutFlow_Massflow] -> AdiabaticManifoldXO2/2
  Conversion_XO2_lambda/1 -> [EngineExhaustManifold_OutletLambda]

== system Supported_and_unsupported_combinations/Engine6/IntakeManifold ==
  Mout : Inport
  inflow : Inport  Port=2
  IsothermalManifoldXO2 : S-Function  FunctionName=orsb_reservoir_isothermal_XO2  Parameters=V , R , Cp , pinit , XO2init ,  EnableBusSupport=off  mask(reservoir isothermal XO2 ){V=41.2801, R=288.4, Cp=1020, pinit=205590, XO2init=0.22}
      mask prompts: V "reservoir volume [l]"; R "gas constant [J/K/kg]"; Cp "fixed pressure spec heat [J/kg/K]"; pinit "initial pressure [Pa]"; XO2init "initial oxygen mass fraction [-]"
      mask help: Isothermal reservoir model with pressure and oxygen mass fraction as internal states.
      mask TabNameString: General ,General ,General ,Initialization ,Initialization
      mask Display:
      | port_label('input', 1, 'min ');
      | port_label('input', 2, 'mout ');
      | port_label('input', 3, 'Tin ');
      | port_label('input', 4, 'O2min ');
      | port_label('output', 1, 'pout ');
      | port_label('output', 2, 'XO2out ');
  Pim : Outport
  XO2out : Outport  Port=2
  outflow : Outport  Port=3
  tag scope: EngineIntakeManifold_OutletPressure=global
  wires:
  Mout/1 -> IsothermalManifoldXO2/2
  IsothermalManifoldXO2/1 -> Pim/1, [EngineIntakeManifold_OutletPressure]
  IsothermalManifoldXO2/2 -> XO2out/1
  inflow/1 -> outflow/1  "flow"
  [MixTotalInFlow_Massflow] -> IsothermalManifoldXO2/1
  [MixTotalInFlow_OxygenFlow] -> IsothermalManifoldXO2/4
  [MixTotalInFlow_MixtureTemperature] -> IsothermalManifoldXO2/3

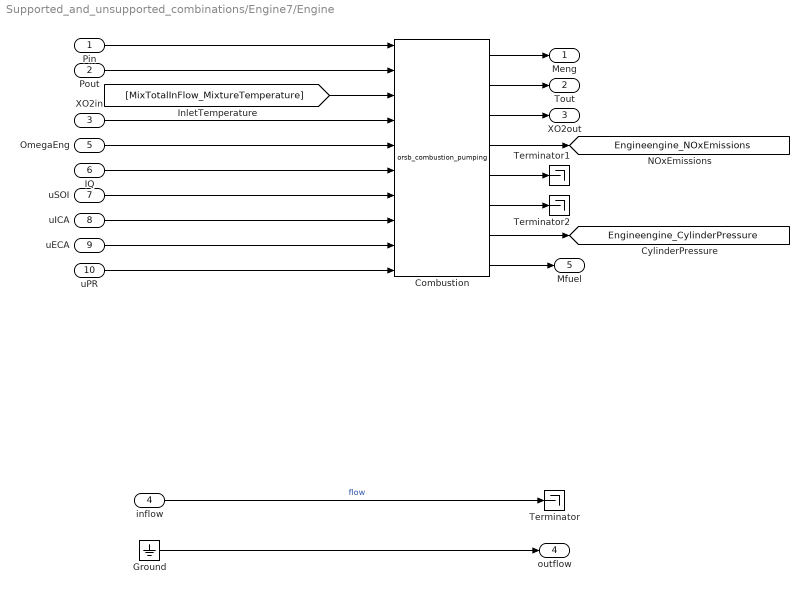
== system Supported_and_unsupported_combinations/Engine7/Engine ==
  Pin : Inport
  Pout : Inport  Port=2
  XO2in : Inport  Port=3
  inflow : Inport  Port=4
  OmegaEng : Inport  Port=5
  IQ : Inport  Port=6
  uSOI : Inport  Port=7
  uICA : Inport  Port=8
  uECA : Inport  Port=9
  uPR : Inport  Port=10
  Combustion : S-Function  FunctionName=orsb_combustion_pumping  Parameters=Displ, CompRatio, Ncyl, ValveMdl, TmpMdl, IgnitMdl, PressMdl, Cp, Cv, port_num_NOx, NOxMdl,  EnableBusSupport=off  mask(combustion_pumping){Displ=12.9, CompRatio=18, Ncyl=6, ValveMdl=[0.00961171539106083 -0.172384589641163], TmpMdl=[-0.025503095647334 0.175522235872159 0.0255043476751577 0.0373865335774022 0], IgnitMdl=[0.484351292851209 0.143524113288744 -0.055676015193126 -0.0109937044135945 -0.025686692856836], PressMdl=[5.48733176777509 -0.092135251339445 -0.0332005633970498 0.773921335537747], Cp=1500, Cv=1200, port_num_NOx=4, NOxMdl=[-0.0710772115732251 13.258266248882 2.53650929146028 -4.98871540780321 18.9690745540948 3.51983329140351 7.35640722696346 -29.5494146545499 -12.7663876549855 -0.0214097840965915 0.143608010417368 -1.21453634962735 0.541720620436424 -0.0774873942784366 -0.515304310267613]}
      mask prompts: Displ "displacement"; CompRatio "compression ratio"; Ncyl "number of cylinders"; ValveMdl "valve model"; TmpMdl "temperature model"; IgnitMdl "ignition model"; PressMdl "pressure model"; port_num_NOx "Model NOx output port number"; NOxMdl "NOx parameters"
      mask help: Combustion development
      mask TabNameString: geometry,geometry,geometry,thermodynamics,thermodynamics,thermodynamics,thermodynamics,thermodynamics,thermodynamics,NOx,NOx
      mask Display:
      | port_label('input', 1, 'Pi');
      | port_label('input', 2, 'Pe');
      | port_label('input', 3, 'Ti');
      | port_label('input', 4, 'O2i');
      | port_label('input', 5, 'Ne');
      | port_label('input', 6, 'iq');
      | port_label('input', 7, 'soi');
      | port_label('input', 8, 'ica');
      | port_label('input', 9, 'eca');
      | port_label('input', 10, 'Prail');
      | port_label('output', 1, 'M');
      | port_label('output', 2, 'Te');
      | port_label('output', 3, 'XO2e');
      | port_label('output', 4, 'NOx');
      | port_label('output', 5, 'lambda');
      | port_label('output', 6, 'phi_ign');
      | port_label('output', 7, 'Pcyl');
      | port_label('output', 8, 'Mf');
  Ground : Ground
  Terminator : Terminator
  Terminator1 : Terminator
  Terminator2 : Terminator
  Meng : Outport
  Tout : Outport  Port=2
  XO2out : Outport  Port=3
  outflow : Outport  Port=4
  Mfuel : Outport  Port=5
  tag scope: Engineengine_CylinderPressure=global, Engineengine_NOxEmissions=global
  wires:
  uSOI/1 -> Combustion/7
  [MixTotalInFlow_MixtureTemperature] -> Combustion/3
  Combustion/4 -> [Engineengine_NOxEmissions]
  XO2in/1 -> Combustion/4
  Combustion/3 -> XO2out/1
  Combustion/2 -> Tout/1
  Pout/1 -> Combustion/2
  Pin/1 -> Combustion/1
  OmegaEng/1 -> Combustion/5
  Ground/1 -> outflow/1
  inflow/1 -> Terminator/1  "flow"
  Combustion/1 -> Meng/1
  Combustion/5 -> Terminator1/1
  Combustion/6 -> Terminator2/1
  Combustion/7 -> [Engineengine_CylinderPressure]
  Combustion/8 -> Mfuel/1
  IQ/1 -> Combustion/6
  uICA/1 -> Combustion/8
  uECA/1 -> Combustion/9
  uPR/1 -> Combustion/10

== system Supported_and_unsupported_combinations/Engine7/ExhaustManifold ==
  Meng : Inport
  Tin : Inport  Port=2
  XO2in : Inport  Port=3
  inflow : Inport  Port=4
  Mfuel : Inport  Port=5
  Add4 : Sum
  AdiabaticManifoldXO2 : S-Function  FunctionName=orsb_reservoir_adiabatic_XO2  Parameters=V , R , Cp , pinit , Tinit , XO2init ,  EnableBusSupport=off  mask(reservoir adiabatic XO2 ){V=50, R=288.4, Cp=1135, pinit=247140, Tinit=720.22, XO2init=0.15}
      mask prompts: V "reservoir volume [l]"; R "gas constant [J/K/kg]"; Cp "fixed pressure spec heat [J/kg/K]"; pinit "initial pressure [Pa]"; Tinit "initial temperature [K]"; XO2init "initial oxygen mass fraction [-]"
      mask help: Adiabatic reservoir model with pressure, temperature, and oxygen mass fraction as internal states.
      mask TabNameString: General ,General ,General ,Initialization ,Initialization ,Initialization
      mask Display:
      | port_label('input', 1, 'min ');
      | port_label('input', 2, 'mout ');
      | port_label('input', 3, 'Tin ');
      | port_label('input', 4, 'O2min ');
      | port_label('output', 1, 'pout ');
      | port_label('output', 2, 'Tout ');
      | port_label('output', 3, 'XO2out ');
  Conversion_XO2_lambda : Fcn  Expr=u(1) / 0.231362 * (1 + 14.59) / (14.59 * (1 - u(1) / 0.231362))+1
  Product2 : Product  RndMeth=Zero
  Saturation : Saturate  UpperLimit=0.2313  LowerLimit=0
  Pout : Outport
  outflow : Outport  Port=2
  tag scope: EngineExhaustManifold_OutletLambda=global, EngineExhaustManifold_OutletOxygenFraction=global, EngineExhaustManifold_OutletPressure=global, EngineExhaustManifold_OutletTemperature=global
  wires:
  Conversion_XO2_lambda/1 -> [EngineExhaustManifold_OutletLambda]
  [FlowSplitterTotalOutFlow_Massflow] -> AdiabaticManifoldXO2/2
  Mfuel/1 -> Add4/1
  inflow/1 -> outflow/1  "flow"
  XO2in/1 -> Product2/2
  AdiabaticManifoldXO2/3 -> [EngineExhaustManifold_OutletOxygenFraction], Saturation/1
  Tin/1 -> AdiabaticManifoldXO2/3
  AdiabaticManifoldXO2/2 -> [EngineExhaustManifold_OutletTemperature]
  AdiabaticManifoldXO2/1 -> [EngineExhaustManifold_OutletPressure], Pout/1
  Meng/1 -> Add4/2
  Product2/1 -> AdiabaticManifoldXO2/4
  Add4/1 -> Product2/1, AdiabaticManifoldXO2/1
  Saturation/1 -> Conversion_XO2_lambda/1

== system Supported_and_unsupported_combinations/Engine7/IntakeManifold ==
  Mout : Inport
  inflow : Inport  Port=2
  IsothermalManifoldXO2 : S-Function  FunctionName=orsb_reservoir_isothermal_XO2  Parameters=V , R , Cp , pinit , XO2init ,  EnableBusSupport=off  mask(reservoir isothermal XO2 ){V=41.2801, R=288.4, Cp=1020, pinit=205590, XO2init=0.22}
      mask prompts: V "reservoir volume [l]"; R "gas constant [J/K/kg]"; Cp "fixed pressure spec heat [J/kg/K]"; pinit "initial pressure [Pa]"; XO2init "initial oxygen mass fraction [-]"
      mask help: Isothermal reservoir model with pressure and oxygen mass fraction as internal states.
      mask TabNameString: General ,General ,General ,Initialization ,Initialization
      mask Display:
      | port_label('input', 1, 'min ');
      | port_label('input', 2, 'mout ');
      | port_label('input', 3, 'Tin ');
      | port_label('input', 4, 'O2min ');
      | port_label('output', 1, 'pout ');
      | port_label('output', 2, 'XO2out ');
  Pim : Outport
  XO2out : Outport  Port=2
  outflow : Outport  Port=3
  tag scope: EngineIntakeManifold_OutletPressure=global
  wires:
  [MixTotalInFlow_MixtureTemperature] -> IsothermalManifoldXO2/3
  [MixTotalInFlow_OxygenFlow] -> IsothermalManifoldXO2/4
  [MixTotalInFlow_Massflow] -> IsothermalManifoldXO2/1
  inflow/1 -> outflow/1  "flow"
  IsothermalManifoldXO2/2 -> XO2out/1
  IsothermalManifoldXO2/1 -> [EngineIntakeManifold_OutletPressure], Pim/1
  Mout/1 -> IsothermalManifoldXO2/2

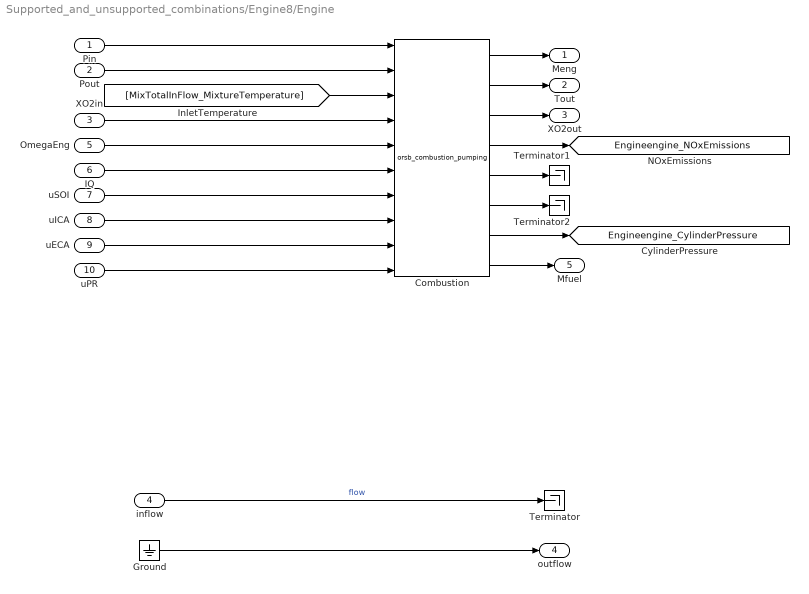
== system Supported_and_unsupported_combinations/Engine8/Engine ==
  Pin : Inport
  Pout : Inport  Port=2
  XO2in : Inport  Port=3
  inflow : Inport  Port=4
  OmegaEng : Inport  Port=5
  IQ : Inport  Port=6
  uSOI : Inport  Port=7
  uICA : Inport  Port=8
  uECA : Inport  Port=9
  uPR : Inport  Port=10
  Combustion : S-Function  FunctionName=orsb_combustion_pumping  Parameters=Displ, CompRatio, Ncyl, ValveMdl, TmpMdl, IgnitMdl, PressMdl, Cp, Cv, port_num_NOx, NOxMdl,  EnableBusSupport=off  mask(combustion_pumping){Displ=12.9, CompRatio=18, Ncyl=6, ValveMdl=[0.00961171539106083 -0.172384589641163], TmpMdl=[-0.025503095647334 0.175522235872159 0.0255043476751577 0.0373865335774022 0], IgnitMdl=[0.484351292851209 0.143524113288744 -0.055676015193126 -0.0109937044135945 -0.025686692856836], PressMdl=[5.48733176777509 -0.092135251339445 -0.0332005633970498 0.773921335537747], Cp=1500, Cv=1200, port_num_NOx=4, NOxMdl=[-0.0710772115732251 13.258266248882 2.53650929146028 -4.98871540780321 18.9690745540948 3.51983329140351 7.35640722696346 -29.5494146545499 -12.7663876549855 -0.0214097840965915 0.143608010417368 -1.21453634962735 0.541720620436424 -0.0774873942784366 -0.515304310267613]}
      mask prompts: Displ "displacement"; CompRatio "compression ratio"; Ncyl "number of cylinders"; ValveMdl "valve model"; TmpMdl "temperature model"; IgnitMdl "ignition model"; PressMdl "pressure model"; port_num_NOx "Model NOx output port number"; NOxMdl "NOx parameters"
      mask help: Combustion development
      mask TabNameString: geometry,geometry,geometry,thermodynamics,thermodynamics,thermodynamics,thermodynamics,thermodynamics,thermodynamics,NOx,NOx
      mask Display:
      | port_label('input', 1, 'Pi');
      | port_label('input', 2, 'Pe');
      | port_label('input', 3, 'Ti');
      | port_label('input', 4, 'O2i');
      | port_label('input', 5, 'Ne');
      | port_label('input', 6, 'iq');
      | port_label('input', 7, 'soi');
      | port_label('input', 8, 'ica');
      | port_label('input', 9, 'eca');
      | port_label('input', 10, 'Prail');
      | port_label('output', 1, 'M');
      | port_label('output', 2, 'Te');
      | port_label('output', 3, 'XO2e');
      | port_label('output', 4, 'NOx');
      | port_label('output', 5, 'lambda');
      | port_label('output', 6, 'phi_ign');
      | port_label('output', 7, 'Pcyl');
      | port_label('output', 8, 'Mf');
  Ground : Ground
  Terminator : Terminator
  Terminator1 : Terminator
  Terminator2 : Terminator
  Meng : Outport
  Tout : Outport  Port=2
  XO2out : Outport  Port=3
  outflow : Outport  Port=4
  Mfuel : Outport  Port=5
  tag scope: Engineengine_CylinderPressure=global, Engineengine_NOxEmissions=global
  wires:
  uPR/1 -> Combustion/10
  uECA/1 -> Combustion/9
  uICA/1 -> Combustion/8
  IQ/1 -> Combustion/6
  Combustion/8 -> Mfuel/1
  Combustion/7 -> [Engineengine_CylinderPressure]
  Combustion/6 -> Terminator2/1
  Combustion/5 -> Terminator1/1
  Combustion/1 -> Meng/1
  inflow/1 -> Terminator/1  "flow"
  Ground/1 -> outflow/1
  OmegaEng/1 -> Combustion/5
  Pin/1 -> Combustion/1
  Pout/1 -> Combustion/2
  Combustion/2 -> Tout/1
  Combustion/3 -> XO2out/1
  XO2in/1 -> Combustion/4
  Combustion/4 -> [Engineengine_NOxEmissions]
  [MixTotalInFlow_MixtureTemperature] -> Combustion/3
  uSOI/1 -> Combustion/7

== system Supported_and_unsupported_combinations/Engine8/ExhaustManifold ==
  Meng : Inport
  Tin : Inport  Port=2
  XO2in : Inport  Port=3
  inflow : Inport  Port=4
  Mfuel : Inport  Port=5
  Add4 : Sum
  AdiabaticManifoldXO2 : S-Function  FunctionName=orsb_reservoir_adiabatic_XO2  Parameters=V , R , Cp , pinit , Tinit , XO2init ,  EnableBusSupport=off  mask(reservoir adiabatic XO2 ){V=50, R=288.4, Cp=1135, pinit=247140, Tinit=720.22, XO2init=0.15}
      mask prompts: V "reservoir volume [l]"; R "gas constant [J/K/kg]"; Cp "fixed pressure spec heat [J/kg/K]"; pinit "initial pressure [Pa]"; Tinit "initial temperature [K]"; XO2init "initial oxygen mass fraction [-]"
      mask help: Adiabatic reservoir model with pressure, temperature, and oxygen mass fraction as internal states.
      mask TabNameString: General ,General ,General ,Initialization ,Initialization ,Initialization
      mask Display:
      | port_label('input', 1, 'min ');
      | port_label('input', 2, 'mout ');
      | port_label('input', 3, 'Tin ');
      | port_label('input', 4, 'O2min ');
      | port_label('output', 1, 'pout ');
      | port_label('output', 2, 'Tout ');
      | port_label('output', 3, 'XO2out ');
  Conversion_XO2_lambda : Fcn  Expr=u(1) / 0.231362 * (1 + 14.59) / (14.59 * (1 - u(1) / 0.231362))+1
  Product2 : Product  RndMeth=Zero
  Saturation : Saturate  UpperLimit=0.2313  LowerLimit=0
  Pout : Outport
  outflow : Outport  Port=2
  tag scope: EngineExhaustManifold_OutletLambda=global, EngineExhaustManifold_OutletOxygenFraction=global, EngineExhaustManifold_OutletPressure=global, EngineExhaustManifold_OutletTemperature=global
  wires:
  Saturation/1 -> Conversion_XO2_lambda/1
  Add4/1 -> AdiabaticManifoldXO2/1, Product2/1
  Product2/1 -> AdiabaticManifoldXO2/4
  Meng/1 -> Add4/2
  AdiabaticManifoldXO2/1 -> Pout/1, [EngineExhaustManifold_OutletPressure]
  AdiabaticManifoldXO2/2 -> [EngineExhaustManifold_OutletTemperature]
  Tin/1 -> AdiabaticManifoldXO2/3
  AdiabaticManifoldXO2/3 -> Saturation/1, [EngineExhaustManifold_OutletOxygenFraction]
  XO2in/1 -> Product2/2
  inflow/1 -> outflow/1  "flow"
  Mfuel/1 -> Add4/1
  [FlowSplitterTotalOutFlow_Massflow] -> AdiabaticManifoldXO2/2
  Conversion_XO2_lambda/1 -> [EngineExhaustManifold_OutletLambda]
